simulink model "LyapunovRedesign"  (R2022a)
settings: Solver=VariableStepAuto  StartTime=0.0  StopTime=10.0  RelTol=1e-3
settings Model: Creator=benja  LastModifiedBy=benja

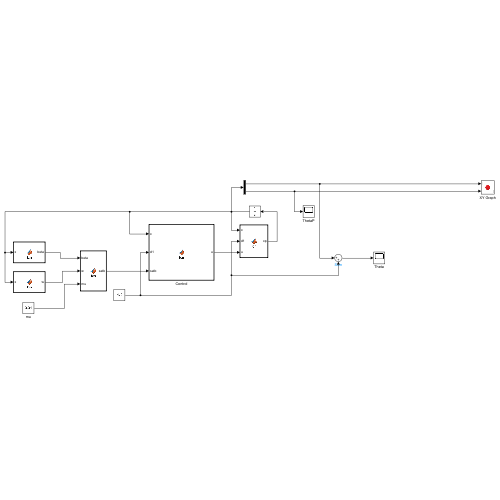
[thumbnail: Simulink's stored preview of the top-level diagram]
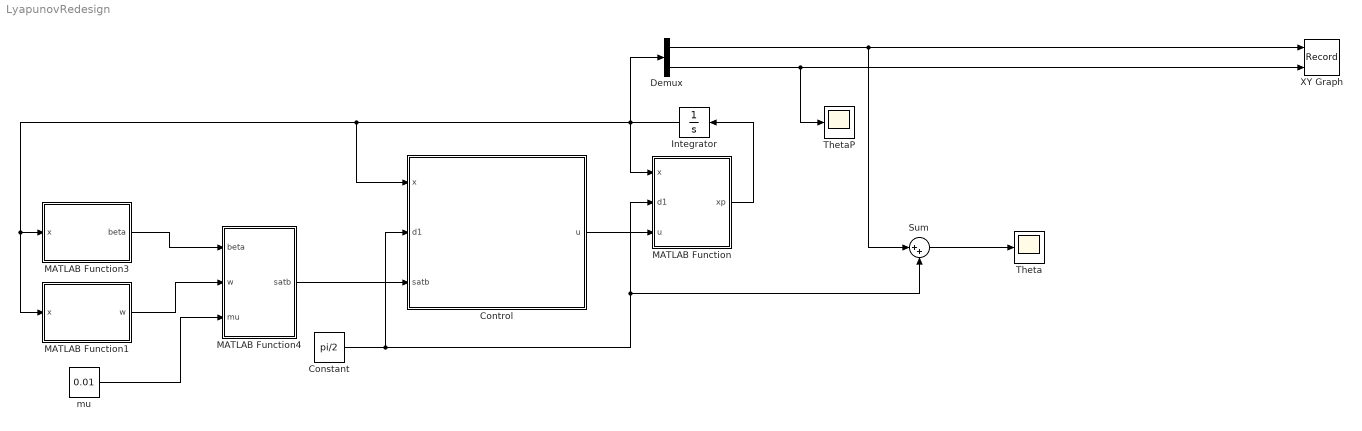
== system LyapunovRedesign ==
  Constant : Constant  Value=pi/2
  Control : MATLAB Function  TreatAsAtomicUnit=on
  Demux : Demux  Outputs=2
  Integrator : Integrator  InitialCondition=[-pi/2 0]
  MATLAB Function : MATLAB Function  TreatAsAtomicUnit=on
  MATLAB Function1 : MATLAB Function  TreatAsAtomicUnit=on
  MATLAB Function3 : MATLAB Function  TreatAsAtomicUnit=on
  MATLAB Function4 : MATLAB Function  TreatAsAtomicUnit=on
  Sum : Sum  Inputs=|++
  Theta : Scope
  ThetaP : Scope
  XY Graph : Record  FileSettingsInternal="{\"entries\":[{\"content\":{\"excelSettings\":{\"content\":{},\"type\":\"Streamout.ExcelSettings\"}},\"type\":\"Streamout.FileSettingStorage\",\"uuid\":\"5d93f739-5142-41f4-af10-d06496daea65\"}],\"packageUris\":[\"http://schema.mathworks.com/mf0/streamout_blocks/R2020a\"],\"version\":\"1.0\"}"  Layout=[1 1]  SignalsInternal="{\"entries\":[{\"content\":{\"signals\":[{\"content\":{\"blockPath\":[\"LyapunovRedesign/XY Graph\"],\"channel\":[],\"dimensions\":[1,1],\"domain\":\"LyapunovRedesign/XY Graph\",\"lineColor\":\"#a2142f\",\"plots\":[1],\"port\":1,\"sid\":[\"\"],\"signalID\":321,\"signalName\":\"Demux:1\"},\"type\":\"RecordBlkView.Signal\",\"uuid\":\"1c3ad78e-0514-486b-9506-4bc0ae7ebb8a\"},{\"content\":{\"blockPath\":[\"LyapunovRedesign/XY Graph\"],\"channel\":[],\"dimensions\":[1,1],\"domain\":\"LyapunovRedesign/XY Graph\",\"lineColor\":\"#139fff\",\"plots\":[1],\"port\":2,\"sid\":[\"\"],\"signalID\":325,\"signalName\":\"Demux:2\"},\"type\":\"RecordBlkView.Signal\",\"uuid\":\"72905eed-c501-41bc-b214-0118e62833d4\"}]},\"type\":\"RecordBlkView.InputSignals\",\"uuid\":\"eb65bb34-53ac-4aaf-b999-a247dc9fb8bc\"}],\"packageUris\":[\"http://schema.mathworks.com/mf0/streamout_blocks/R2020a\"],\"version\":\"1.0\"}"  VisualizationBindings="{\"xyplotplugin\":{\"info\":[{\"series\":[{\"bindingParametersList\":[{\"parameter\":\"X-Axis\",\"signalID\":321,\"signalName\":\"Demux:1\"},{\"parameter\":\"Y-Axis\",\"signalID\":325,\"signalName\":\"Demux:2\"}],\"seriesID\":23706}],\"subplotID\":1}]}}"  CompatibilityTag=XY
  mu : Constant  Value=0.01
  wires:
  MATLAB Function/1(xp) -> Integrator/1
  Integrator/1 -> Control/1(x), MATLAB Function1/1(x), MATLAB Function3/1(x), MATLAB Function/1(x), Demux/1
  Constant/1 -> Sum/2, MATLAB Function/2(d1), Control/2(d1)
  mu/1 -> MATLAB Function4/3(mu)
  MATLAB Function3/1(beta) -> MATLAB Function4/1(beta)
  MATLAB Function4/1(satb) -> Control/3(satb)
  Control/1(u) -> MATLAB Function/3(u)
  MATLAB Function1/1(w) -> MATLAB Function4/2(w)
  Demux/2 -> XY Graph/2, ThetaP/1
  Demux/1 -> XY Graph/1, Sum/1
  Sum/1 -> Theta/1

== matlab function LyapunovRedesign/MATLAB Function1 ==
  data: x input; w output
function w = fcn(x)

w = x(1)+x(2)

== matlab function LyapunovRedesign/MATLAB Function ==
  data: x input; d1 input; u input; xp output
function xp = fcn(x,d1,u)

b0 = 0.01
c = 0.5

x1p = x(2);
x2p = -sin( x(1) + d1 ) - b0*x(2) + c*u;

xp = [x1p, x2p]

== matlab function LyapunovRedesign/Control ==
  data: u output; x input; d1 input; satb input
function u = fcn(x,d1,satb)
ch = 1.25
% u = 0.8*(cos(x(1)) - x(1) - 2*x(2)) - satb;
k1 = 1
k2 = 2
u = (1/ch)*(sin(x(1) + d1) -k1*x(1) - k2*x(2)) - satb;

== matlab function LyapunovRedesign/MATLAB Function3 ==
  data: x input; beta output
function beta = fcn(x)    
    beta = 2.4*abs(x(1)) + 2.8*abs(x(2)) + 1.5;

== matlab function LyapunovRedesign/MATLAB Function4 ==
  data: beta input; w input; satb output; mu input
function satb  = fcn(beta, w, mu)


condicion = beta*abs(w);

satb = 0

if condicion > mu
    satb = beta*(w/abs(w));
end

if condicion <= mu
    satb = beta^2*(w/mu);
end
